simulink model "A14_Servoachse_Kaskade_i"  (R2017b)
settings: Solver=ode45  StartTime=0.0  StopTime=5  FixedStep=0.001  RelTol=1e-3  EnableMultiTasking=on
values from neighbouring files (symbols this model uses):
  CM = 7.1e-7    (= 7.1e-07)    [A10_Konstanten.m]    (also in A13_Konstanten.m; A14_Konstanten.m; A16_Konstanten.m)
  JR = 1.32e-6    (= 1.32e-06)    [A10_Konstanten.m]    (also in A13_Konstanten.m; A14_Konstanten.m; A16_Konstanten.m; A9_Konstanten.m = 0.004)
  KM = 38.4e-3    (= 0.0384)    [A10_Konstanten.m]    (also in A13_Konstanten.m; A14_Konstanten.m; A16_Konstanten.m)
  KN = 1/(2*pi*KM)    (= 4.14465997635)    [A10_Konstanten.m]    (also in A13_Konstanten.m; A14_Konstanten.m; A16_Konstanten.m)
  LA = 4.64e-4    (= 0.000464)    [A10_Konstanten.m]    (also in A13_Konstanten.m; A14_Konstanten.m; A16_Konstanten.m)
  RA = 4.99    [A10_Konstanten.m]    (also in A13_Konstanten.m; A14_Konstanten.m; A16_Konstanten.m)
  Tisens = 2e-5    (= 2e-05)    [A14_Konstanten.m]
  TPWM = 2e-5    (= 2e-05)    [A14_Konstanten.m]
  Umax = 24    [A10_Konstanten.m]    (also in A13_Konstanten.m; A14_Konstanten.m; A16_Konstanten.m; A17_Konstanten.m = 120)
undefined symbols (not defined in the file or in its folder): sigbuilder_block
libraries: simulink x2
settings Model: Creator=jbaur  LastModifiedBy=jbaur
settings DataIOCC: ExternalInput=X1  SaveFormat=StructureWithTime  SignalLoggingName=sigsOut
settings OptimizationCC: DefaultParameterBehavior=Inlined  InlineInvariantSignals=on  BufferReuse=off  ExpressionDepthLimit=2147483647  InitFltsAndDblsToZero=on  LifeSpan=inf
settings DebuggingCC: SaveWithParameterizedLinksMsg=none  SignalResolutionControl=TryResolveAllWithWarning  MultiTaskDSMMsg=warning  MultiTaskCondExecSysMsg=none  StateNameClashWarn=warning  InitInArrayFormatMsg=none  SFUnexpectedBacktrackingDiag=warning  SFNoUnconditionalDefaultTransitionDiag=warning  SFExecutionAtInitializationDiag=none
settings HardwareCC: ProdBitPerPointer=32  ProdBitPerSizeT=32  ProdBitPerPtrDiffT=32  ProdLargestAtomicFloat=None  ProdIntDivRoundTo=Undefined  ProdEndianess=Unspecified  ProdWordSize=32  ProdHWDeviceType=32-bit Generic  TargetUnknown=on
settings ModelReferenceCC: PropagateSignalLabelsOutOfModel=off
settings CodeAppCC: StateflowObjectComments=on
settings GRTTargetCC: TargetFcnLib=ansi_tfl_tmw.mat  TargetLangStandard=C89/C90 (ANSI)  ModelReferenceCompliant=off  GeneratePreprocessorConditionals=Disable all  CombineOutputUpdateFcns=off  MatFileLogging=off  GRTInterface=on
settings ConfigComp: CovMetricSettings=dw  CovHtmlReporting=on  CovSaveCumulativeToWorkspaceVar=on  CovSaveSingleToWorkspaceVar=on  CovExternalEMLEnable=off  CovSFcnEnable=off

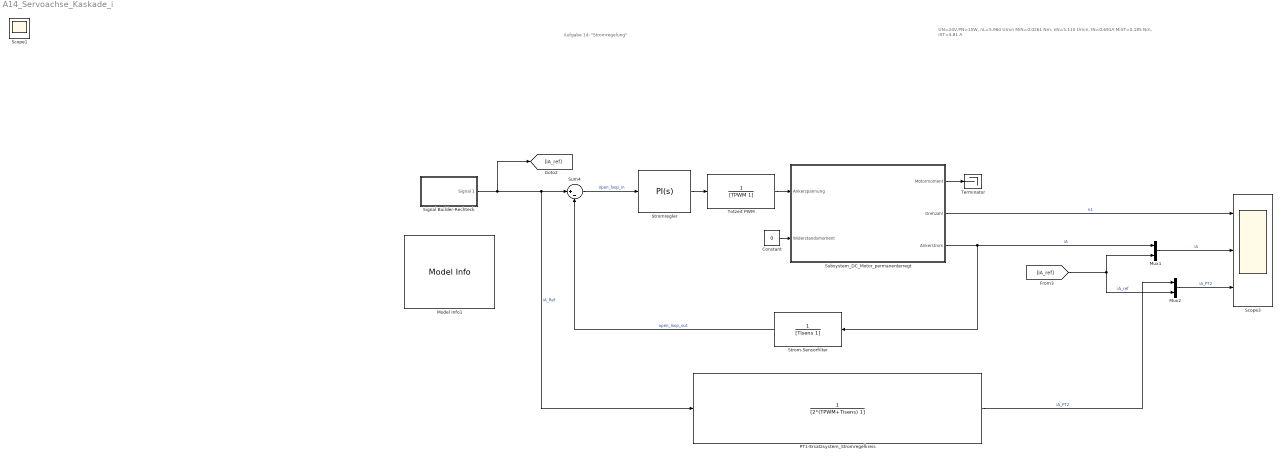
== system A14_Servoachse_Kaskade_i ==
  note: UN=24V,PN=15W, nL=5.960 Umin
      | MiN=0.0261 Nm, nN=5.110 Umin, IN=0.691A
      | MiST=0.185 Nm, IST=4.81 A
  note: Aufgabe 14: "Stromregelung"
  Constant : Constant  Value=0
  Model Info1 : simulink/Model-Wide Utilities/Model Info  Frame=on  DisplayStringWithTags=|  HorizontalTextAlignment=Left  LeftAlignmentValue=0.02
      | Bewegungsprofil:
      | ------------------------
      | Tmax = 1s
      | smax = 0,5m
      | vmax = 1 m/s
      | amax = 2 m/s^2
  Mux1 : Mux  Inputs=2
  Mux2 : Mux  Inputs=2
  PT1-Ersatzsystem_Stromregelkreis : TransferFcn  Denominator=[2*(TPWM+Tisens) 1]
  Scope3 : Scope  NumInputPorts=3
  Signal Builder-Rechteck : Subsystem  Tag=STV Subsys  LoadFcn=sigbuilder_block('load');  StartFcn=sigbuilder_block('start');  StopFcn=sigbuilder_block('stop');  ClipboardFcn=sigbuilder_block('clipboard');  mask(Sigbuilder block){tuvar=[0:10]}
      mask help: Create and generate interchangeable groups of signals whose waveforms are piecewise linear.
      mask init:
      | if ~strcmp(get_param(bdroot(gcbh),'SimulationStatus'),'stopped') tuvar = sigbuilder_block('maskInit'); end
      settings: CopyFcn=sigbuilder_block('copy');  DeleteFcn=sigbuilder_block('delete');  ModelCloseFcn=sigbuilder_block('modelClose');  PreSaveFcn=sigbuilder_block('preSave');  PauseFcn=sigbuilder_block('pause')  ContinueFcn=sigbuilder_block('continue')  NameChangeFcn=sigbuilder_block('namechange');  OpenFcn=sigbuilder_block('open',[437.25 199.5 550.5 399.75 ]);  CloseFcn=sigbuilder_block('close');
      mask Display: plot(0, 0, 100, 100,[2, 2, 32, 32, 2], [68, 8, 8, 68, 68],[32, 2], [38, 38], [32, 19, 2],[53, 60, 44], [32, 17, 17, 2],[16, 16, 31, 31]);txt = getActiveGroup(gcbh);text(2, 100, txt,'verticalAlignment', 'top');
  Strom-Sensorfilter : TransferFcn  Denominator=[Tisens 1]
  Stromregler : simulink/Continuous/PID Controller  Controller=PI  TimeDomain=Continuous-time  SampleTime=-1  IntegratorMethod=Forward Euler  FilterMethod=Forward Euler  Form=Ideal  UseFilter=on  ControllerParametersSource=internal  P=1  I=1  D=-0.00136816077946148  N=3731.68343054543  InitialConditionSource=internal  InitialConditionForIntegrator=0  InitialConditionForFilter=0  ExternalReset=none  LimitOutput=off  UpperSaturationLimit=Umax  LowerSaturationLimit=-Umax  LinearizeAsGain=on  AntiWindupMode=clamping  Kb=1  TrackingMode=off  Kt=1  PParamMin=[]  PParamMax=[]  IParamMin=[]  IParamMax=[]  DParamMin=[]  DParamMax=[]  NParamMin=[]  NParamMax=[]  KbParamMin=[]  KbParamMax=[]  KtParamMin=[]  KtParamMax=[]  POutMin=[]  POutMax=[]  IOutMin=[]  IOutMax=[]  DOutMin=[]  DOutMax=[]  NOutMin=[]  NOutMax=[]  KbOutMin=[]  KbOutMax=[]  KtOutMin=[]  KtOutMax=[]  IntegratorOutMin=[]  IntegratorOutMax=[]  FilterOutMin=[]  FilterOutMax=[]  SumOutMin=[]  SumOutMax=[]  SumI1OutMin=[]  SumI1OutMax=[]  SumI2OutMin=[]  SumI2OutMax=[]  SumI3OutMin=[]  SumI3OutMax=[]  SumDOutMin=[]  SumDOutMax=[]  SaturationOutMin=[]  SaturationOutMax=[]  IntegratorContinuousStateAttributes=''  IntegratorStateMustResolveToSignalObject=off  IntegratorRTWStateStorageClass=Auto  FilterContinuousStateAttributes=''  FilterStateMustResolveToSignalObject=off  FilterRTWStateStorageClass=Auto  DifferentiatorICPrevScaledInput=0  DifferentiatorOutMin=[]  DifferentiatorOutMax=[]  InitialConditionSetting=State (most efficient)  FilterDiffOutCoefMin=[]  FilterDiffOutCoefMax=[]  SumDenOutMin=[]  SumDenOutMax=[]  SumNumOutMin=[]  SumNumOutMax=[]  ReciprocalOutMin=[]  ReciprocalOutMax=[]  DivideOutMin=[]  DivideOutMax=[]  TunerSelectOption=Transfer Function Based (PID Tuner App)
  Subsystem_DC_Motor_permanenterregt : Subsystem
  Sum4 : Sum  Inputs=|+-
  Terminator : Terminator
  Totzeit PWM : TransferFcn  Denominator=[TPWM 1]
  Scope1 : Scope
  wires:
  Sum4/1 -> Stromregler/1  "open_loop_in"
  Stromregler/1 -> Totzeit PWM/1
  Signal Builder-Rechteck/1(Signal 1) -> [iA_ref], PT1-Ersatzsystem_Stromregelkreis/1, Sum4/1  "iA_Ref"
  Subsystem_DC_Motor_permanenterregt/1(Motormoment) -> Terminator/1
  Strom-Sensorfilter/1 -> Sum4/2  "open_loop_out"
  Totzeit PWM/1 -> Subsystem_DC_Motor_permanenterregt/1(Ankerspannung)
  Constant/1 -> Subsystem_DC_Motor_permanenterregt/2(Widerstandsmoment)
  Subsystem_DC_Motor_permanenterregt/3(Ankerstrom) -> Mux1/1, Strom-Sensorfilter/1  "iA"
  Mux1/1 -> Scope3/2  "iA"
  [iA_ref] -> Mux2/2, Mux1/2  "iA_ref"
  Mux2/1 -> Scope3/3  "iA_PT2"
  Subsystem_DC_Motor_permanenterregt/2(Drehzahl) -> Scope3/1  "n1"
  PT1-Ersatzsystem_Stromregelkreis/1 -> Mux2/1  "iA_PT2"

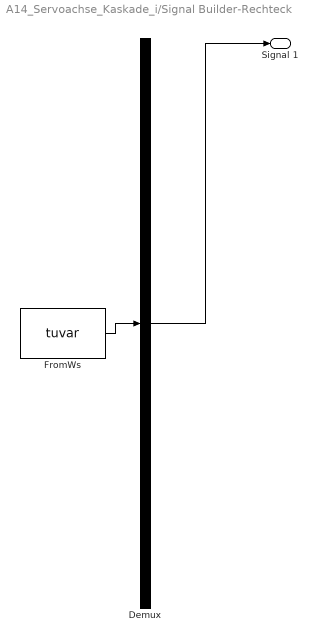
== system A14_Servoachse_Kaskade_i/Signal Builder-Rechteck ==
  Demux : Demux  Tag=STV Demux  Outputs=1
  FromWs : FromWorkspace  Tag=STV FromWs  VariableName=tuvar  SampleTime=0
      SigBuilderData=|
      | common.afterFinalStr = 'Extrapolate'
      | common.sampleTime = 0
      | dataSet.timeRange = [0 5]
      | dataSet.name = 'Group 1'
      | sbobj.Groups.Name = 'Group 1'
      | sbobj.Groups.Signals.Name = 'Signal 1'
      | sbobj.Groups.Signals.XData = [0 1 1 1.5 1.5 2 2 5]
      | sbobj.Groups.Signals.YData = [0 0 0.7 0.7 -0.7 -0.7 0 0]
      | sbobj.Groups.TimeRange = [0 5]
  Signal 1 : Outport  Tag=STV Outport
  wires:
  Demux/1 -> Signal 1/1
  FromWs/1 -> Demux/1

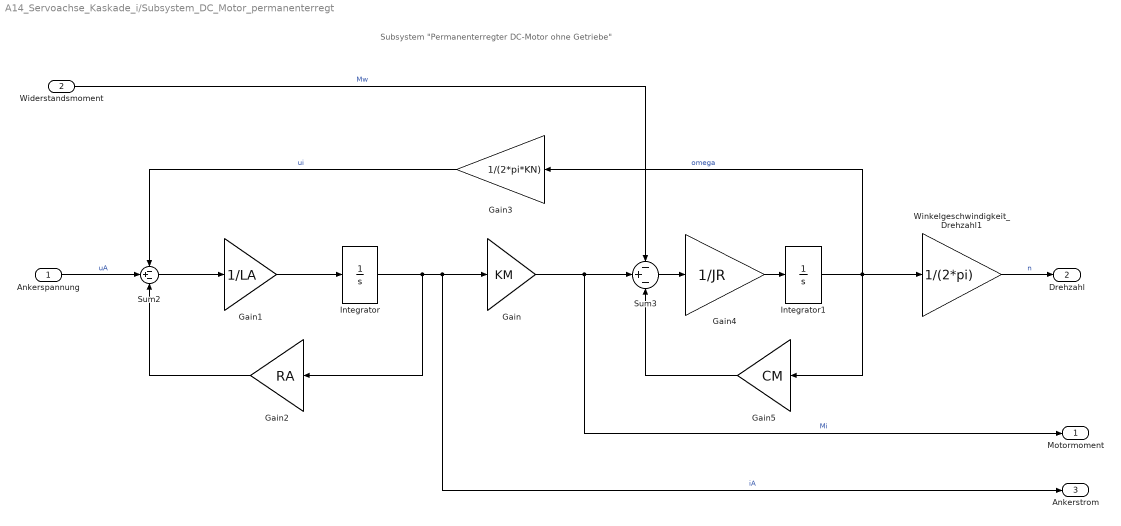
== system A14_Servoachse_Kaskade_i/Subsystem_DC_Motor_permanenterregt ==
  note: Subsystem "Permanenterregter DC-Motor ohne Getriebe"
  Ankerspannung : Inport
  Widerstandsmoment : Inport  Port=2
  Gain : Gain  Gain=KM
  Gain1 : Gain  Gain=1/LA
  Gain2 : Gain  Gain=RA
  Gain3 : Gain  Gain=1/(2*pi*KN)
  Gain4 : Gain  Gain=1/JR
  Gain5 : Gain  Gain=CM
  Integrator : Integrator
  Integrator1 : Integrator
  Sum2 : Sum  Inputs=-+-
  Sum3 : Sum  Inputs=-+-
  Winkelgeschwindigkeit_Drehzahl1 : Gain  Gain=1/(2*pi)
  Motormoment : Outport
  Drehzahl : Outport  Port=2
  Ankerstrom : Outport  Port=3
  wires:
  Ankerspannung/1 -> Sum2/2  "uA"
  Gain/1 -> Sum3/2, Motormoment/1  "Mi"
  Winkelgeschwindigkeit_Drehzahl1/1 -> Drehzahl/1  "n"
  Sum2/1 -> Gain1/1
  Gain1/1 -> Integrator/1
  Integrator/1 -> Gain2/1, Ankerstrom/1, Gain/1  "iA"
  Sum3/1 -> Gain4/1
  Gain4/1 -> Integrator1/1
  Integrator1/1 -> Gain3/1, Winkelgeschwindigkeit_Drehzahl1/1, Gain5/1  "omega"
  Gain5/1 -> Sum3/3
  Gain2/1 -> Sum2/3
  Widerstandsmoment/1 -> Sum3/1  "Mw"
  Gain3/1 -> Sum2/1  "ui"
